simulink model "LEDLC"  (R2022b)
settings: Solver=FixedStepAuto  StartTime=0.0  StopTime=10.0  FixedStep=1  RelTol=1e-3
libraries: simulink x16
settings Model: Creator=yuzehong  LastModifiedBy=yuzehong
settings OptimizationCC: DefaultParameterBehavior=Inlined  BufferReuse=off  GlobalBufferReuse=off  ExpressionFolding=off  EnableMemcpy=off  PassReuseOutputArgsAs=Individual arguments  NoFixptDivByZeroProtection=on  EfficientFloat2IntCast=on  OptimizeDataStoreBuffers=off  BusAssignmentInplaceUpdate=off  OptimizationLevel=level0  EfficientTunableParamExpr=on
settings DebuggingCC: ParameterTunabilityLossMsg=error  UnconnectedInputMsg=warning  UnconnectedOutputMsg=warning  UnconnectedLineMsg=warning
settings ModelReferenceCC: EnableRefExpFcnMdlSchedulingChecks=on
settings SFSimCC: MATLABDynamicMemAlloc=off
settings RTWCC: Description=Embedded Coder  SystemTargetFile=ert.tlc  GenCodeOnly=on  TemplateMakefile=ert_default_tmf  DLArmComputeVersion=19.05
settings CodeAppCC: GenerateComments=off  IgnoreCustomStorageClasses=off  OperatorAnnotations=on  SimulinkDataObjDesc=on  SFDataObjDesc=on  SimulinkBlockComments=off
settings ERTTargetCC: TargetLangStandard=C99 (ISO)  GenerateSampleERTMain=on  CodeInterfacePackaging=Reusable function  InlinedParameterPlacement=NonHierarchical  ERTCustomFileTemplate=example_file_process.tlc
settings ConfigComp: DVMaxProcessTime=3600  DVTestSuiteOptimization=Auto  DVDetectOutOfBounds=on  DVSaveHarnessModel=on  DVModelReferenceHarness=on

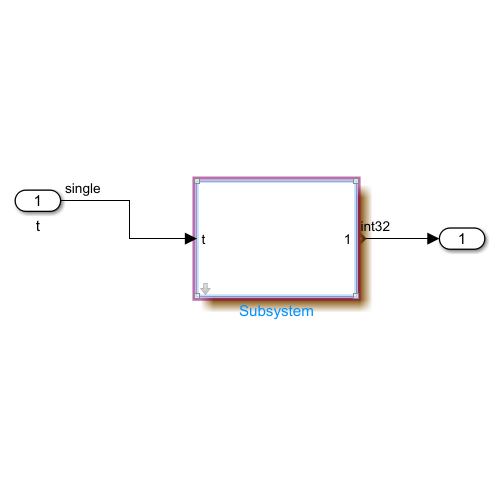
[thumbnail: Simulink's stored preview of the top-level diagram]
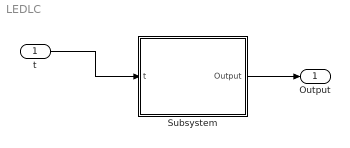
== system LEDLC ==
  t : Inport
  Subsystem : Subsystem  mask{length=64, id=3142}
      mask DialogControl ParameterGroupVar Prompt: 参数
  Output : Outport
  wires:
  t/1 -> Subsystem/1(t)
  Subsystem/1(Output) -> Output/1

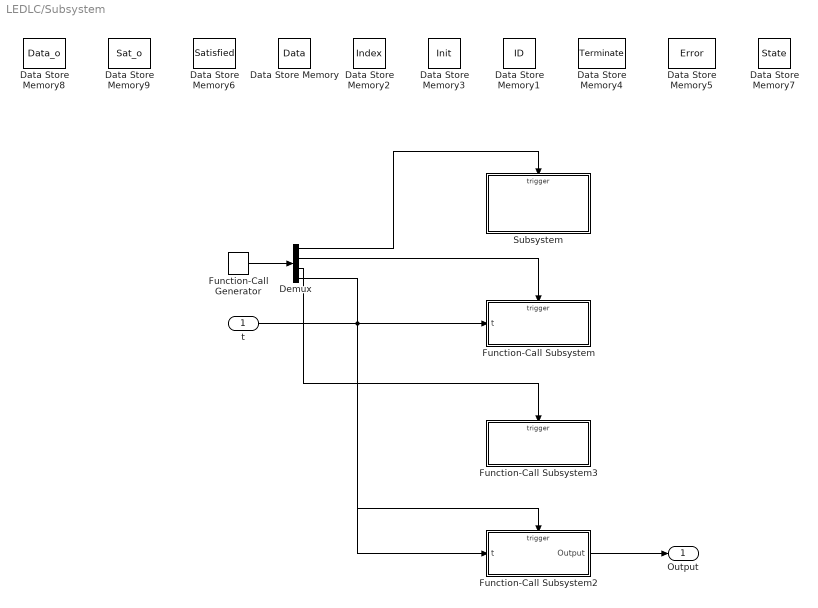
== system LEDLC/Subsystem ==
  t : Inport
  Data Store Memory : DataStoreMemory  DataStoreName=Data  WriteAfterWriteMsg=warning  ShowAdditionalParam=off  OutDataTypeStr=single  Dimensions=length
  Data Store Memory1 : DataStoreMemory  DataStoreName=ID  WriteAfterWriteMsg=warning  ShowAdditionalParam=off  OutDataTypeStr=int32
  Data Store Memory2 : DataStoreMemory  DataStoreName=Index  WriteAfterWriteMsg=warning  ShowAdditionalParam=off  OutDataTypeStr=int32
  Data Store Memory3 : DataStoreMemory  DataStoreName=Init  WriteAfterWriteMsg=warning  ShowAdditionalParam=off  OutDataTypeStr=int32
  Data Store Memory4 : DataStoreMemory  DataStoreName=Terminate  WriteAfterWriteMsg=warning  ShowAdditionalParam=off  OutDataTypeStr=int32
  Data Store Memory5 : DataStoreMemory  DataStoreName=Error  WriteAfterWriteMsg=warning  ShowAdditionalParam=off  OutDataTypeStr=int32
  Data Store Memory6 : DataStoreMemory  DataStoreName=Satisfied  WriteAfterWriteMsg=warning  ShowAdditionalParam=off  OutDataTypeStr=int32  Dimensions=length
  Data Store Memory7 : DataStoreMemory  DataStoreName=State  WriteAfterWriteMsg=warning  ShowAdditionalParam=off
  Data Store Memory8 : DataStoreMemory  DataStoreName=Data_o  WriteAfterWriteMsg=warning  ShowAdditionalParam=off  OutDataTypeStr=single  Dimensions=length
  Data Store Memory9 : DataStoreMemory  DataStoreName=Sat_o  WriteAfterWriteMsg=warning  ShowAdditionalParam=off  OutDataTypeStr=int32  Dimensions=length
  Demux : Demux
  Function-Call Generator : simulink/Ports & Subsystems/Function-Call Generator  sample_time=-1  numberOfIterations=1  DisallowWideOutput=off
  Function-Call Subsystem : Subsystem  TreatAsAtomicUnit=on
  Function-Call Subsystem2 : Subsystem  TreatAsAtomicUnit=on
  Function-Call Subsystem3 : Subsystem  TreatAsAtomicUnit=on
  Subsystem : Subsystem
  Output : Outport
  wires:
  Function-Call Generator/1 -> Demux/1
  Demux/1 -> Subsystem/Trigger
  t/1 -> Function-Call Subsystem/1(t), Function-Call Subsystem2/1(t)
  Demux/3 -> Function-Call Subsystem3/Trigger
  Function-Call Subsystem2/1(Output) -> Output/1
  Demux/4 -> Function-Call Subsystem2/Trigger
  Demux/2 -> Function-Call Subsystem/Trigger

== system LEDLC/Subsystem/Function-Call Subsystem ==
  t : Inport
  function : TriggerPort  TriggerType=function-call  VariantControl=(inherit)
  Demux : Demux  Outputs=3
  Function-Call Generator : simulink/Ports & Subsystems/Function-Call Generator  sample_time=-1  numberOfIterations=1  DisallowWideOutput=off
  Function-Call Subsystem : Subsystem  TreatAsAtomicUnit=on
  If Action Subsystem1 : Subsystem  TreatAsAtomicUnit=on
  Subsystem : Subsystem
  wires:
  Function-Call Generator/1 -> Demux/1
  Demux/3 -> If Action Subsystem1/Trigger
  Demux/1 -> Function-Call Subsystem/Trigger
  Demux/2 -> Subsystem/Trigger
  t/1 -> If Action Subsystem1/1(Inport)

== system LEDLC/Subsystem/Function-Call Subsystem2 ==
  t : Inport
  function : TriggerPort  TriggerType=function-call  VariantControl=(inherit)
  Data Store Read : DataStoreRead  DataStoreName=Terminate  IndexOptions=Index vector (dialog)  Indices=1  OutputSizes=1
  If : If  IfExpression=u1 == 0
  If Action Subsystem : Subsystem  TreatAsAtomicUnit=on
  Terminator : Terminator
  Output : Outport
  wires:
  Data Store Read/1 -> If/1
  If/1 -> Terminator/1
  If/2 -> If Action Subsystem/Action
  t/1 -> If Action Subsystem/1(t)
  If Action Subsystem/1(Output1) -> Output/1

== system LEDLC/Subsystem/Function-Call Subsystem3 ==
  function : TriggerPort  TriggerType=function-call  VariantControl=(inherit)
  Demux : Demux  Outputs=2
  Function-Call Generator : simulink/Ports & Subsystems/Function-Call Generator  sample_time=-1  numberOfIterations=1  DisallowWideOutput=off
  Function-Call Subsystem : Subsystem  TreatAsAtomicUnit=on
  Subsystem : Subsystem
  wires:
  Function-Call Generator/1 -> Demux/1
  Demux/1 -> Function-Call Subsystem/Trigger
  Demux/2 -> Subsystem/Trigger

== system LEDLC/Subsystem/Subsystem ==
  function : TriggerPort  TriggerType=function-call  VariantControl=(inherit)
  Data Store Read1 : DataStoreRead  DataStoreName=Init  IndexOptions=Index vector (dialog)  Indices=1  OutputSizes=1
  If Action Subsystem1 : Subsystem  TreatAsAtomicUnit=on
  If1 : If  IfExpression=u1 == 0
  Terminator : Terminator
  wires:
  Data Store Read1/1 -> If1/1
  If1/1 -> If Action Subsystem1/Action
  If1/2 -> Terminator/1

== system LEDLC/Subsystem/Function-Call Subsystem/Function-Call Subsystem ==
  function : TriggerPort  TriggerType=function-call  VariantControl=(inherit)
  Constant : Constant  Value=-1  OutDataTypeStr=int32
  Data Store Write : DataStoreWrite  DataStoreName=Index  IndexOptions=Index vector (dialog)  Indices=1  OutputSizes=1
  wires:
  Constant/1 -> Data Store Write/1

== system LEDLC/Subsystem/Function-Call Subsystem/If Action Subsystem1 ==
  Inport : Inport
  function : TriggerPort  TriggerType=function-call  VariantControl=(inherit)
  Data Store Read2 : DataStoreRead  DataStoreName=Index  IndexOptions=Index vector (dialog)  Indices=1  OutputSizes=1
  If : If  IfExpression=u1 ~= -1
  If Action Subsystem : Subsystem  TreatAsAtomicUnit=on
  Terminator : Terminator
  wires:
  Data Store Read2/1 -> If/1
  If/1 -> If Action Subsystem/Action
  If/2 -> Terminator/1
  Inport/1 -> If Action Subsystem/1(t)

== system LEDLC/Subsystem/Function-Call Subsystem/Subsystem ==
  function : TriggerPort  TriggerType=function-call  VariantControl=(inherit)
  For Iterator Subsystem : Subsystem  TreatAsAtomicUnit=on

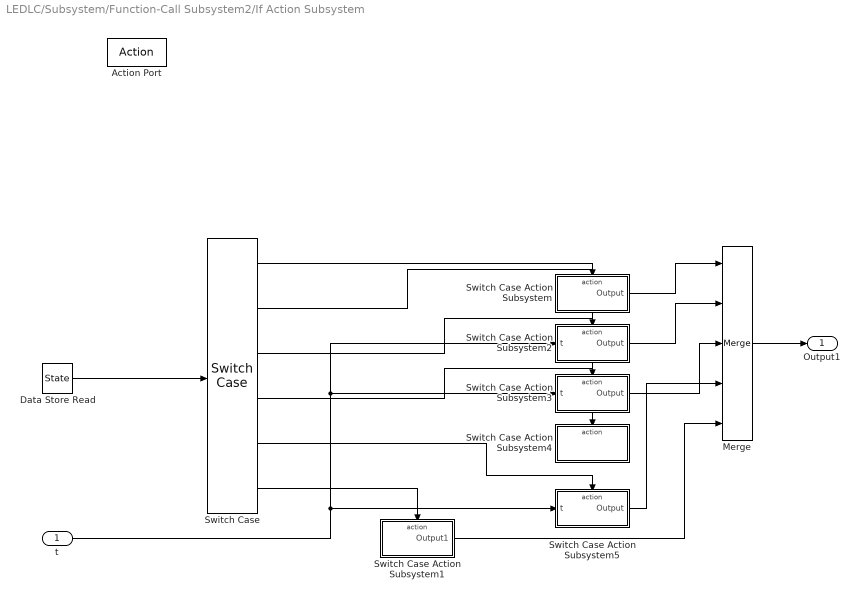
== system LEDLC/Subsystem/Function-Call Subsystem2/If Action Subsystem ==
  t : Inport
  Action Port : ActionPort  ActionPortLabel=else
  Data Store Read : DataStoreRead  DataStoreName=State  IndexOptions=Index vector (dialog)  Indices=1  OutputSizes=1
  Merge : Merge  Inputs=5
  Switch Case : SwitchCase  CaseConditions={0,1,2,3,4}
  Switch Case Action Subsystem : Subsystem  TreatAsAtomicUnit=on
  Switch Case Action Subsystem1 : Subsystem  TreatAsAtomicUnit=on
  Switch Case Action Subsystem2 : Subsystem  TreatAsAtomicUnit=on
  Switch Case Action Subsystem3 : Subsystem  TreatAsAtomicUnit=on
  Switch Case Action Subsystem4 : Subsystem  TreatAsAtomicUnit=on
  Switch Case Action Subsystem5 : Subsystem  TreatAsAtomicUnit=on
  Output1 : Outport  OutDataTypeStr=int32
  wires:
  Data Store Read/1 -> Switch Case/1
  Switch Case/1 -> Switch Case Action Subsystem/Action
  Switch Case/6 -> Switch Case Action Subsystem1/Action
  t/1 -> Switch Case Action Subsystem5/1(t), Switch Case Action Subsystem3/1(t), Switch Case Action Subsystem2/1(t)
  Switch Case/2 -> Switch Case Action Subsystem2/Action
  Switch Case Action Subsystem/1(Output) -> Merge/1
  Merge/1 -> Output1/1
  Switch Case Action Subsystem1/1(Output1) -> Merge/5
  Switch Case Action Subsystem2/1(Output) -> Merge/2
  Switch Case/3 -> Switch Case Action Subsystem3/Action
  Switch Case Action Subsystem3/1(Output) -> Merge/3
  Switch Case/4 -> Switch Case Action Subsystem4/Action
  Switch Case/5 -> Switch Case Action Subsystem5/Action
  Switch Case Action Subsystem5/1(Output) -> Merge/4

== system LEDLC/Subsystem/Function-Call Subsystem3/Function-Call Subsystem ==
  function : TriggerPort  TriggerType=function-call  VariantControl=(inherit)
  Data Store Read : DataStoreRead  DataStoreName=Terminate  IndexOptions=Index vector (dialog)  Indices=1  OutputSizes=1
  If : If
  If Action Subsystem1 : Subsystem  TreatAsAtomicUnit=on
  Terminator : Terminator
  wires:
  Data Store Read/1 -> If/1
  If/2 -> If Action Subsystem1/Action
  If/1 -> Terminator/1

== system LEDLC/Subsystem/Function-Call Subsystem3/Subsystem ==
  function : TriggerPort  TriggerType=function-call  VariantControl=(inherit)
  For Iterator Subsystem : Subsystem  TreatAsAtomicUnit=on

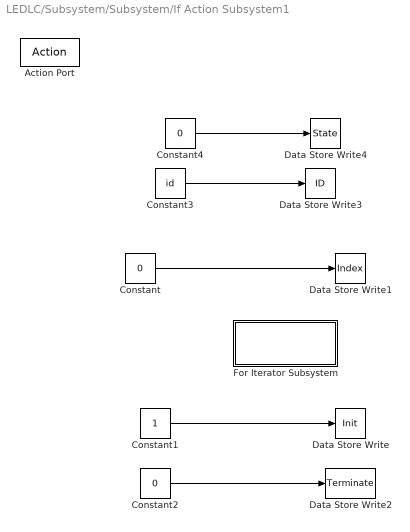
== system LEDLC/Subsystem/Subsystem/If Action Subsystem1 ==
  Action Port : ActionPort  ActionPortLabel=if(u1 == 0)
  Constant : Constant  Value=0  OutDataTypeStr=int32
  Constant1 : Constant  OutDataTypeStr=int32
  Constant2 : Constant  Value=0  OutDataTypeStr=int32
  Constant3 : Constant  Value=id  OutDataTypeStr=int32
  Constant4 : Constant  Value=0  OutDataTypeStr=int32
  Data Store Write : DataStoreWrite  DataStoreName=Init  IndexOptions=Index vector (dialog)  Indices=1  OutputSizes=1
  Data Store Write1 : DataStoreWrite  DataStoreName=Index  IndexOptions=Index vector (dialog)  Indices=1  OutputSizes=1
  Data Store Write2 : DataStoreWrite  DataStoreName=Terminate  IndexOptions=Index vector (dialog)  Indices=1  OutputSizes=1
  Data Store Write3 : DataStoreWrite  DataStoreName=ID  IndexOptions=Index vector (dialog)  Indices=1  OutputSizes=1
  Data Store Write4 : DataStoreWrite  DataStoreName=State  IndexOptions=Index vector (dialog)  Indices=1  OutputSizes=1
  For Iterator Subsystem : Subsystem  TreatAsAtomicUnit=on
  wires:
  Constant/1 -> Data Store Write1/1
  Constant1/1 -> Data Store Write/1
  Constant2/1 -> Data Store Write2/1
  Constant3/1 -> Data Store Write3/1
  Constant4/1 -> Data Store Write4/1

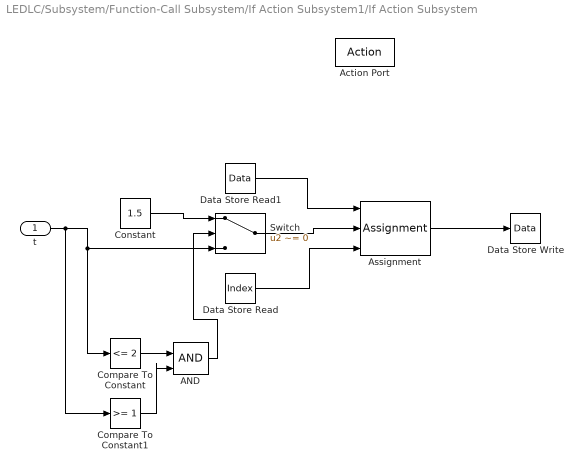
== system LEDLC/Subsystem/Function-Call Subsystem/If Action Subsystem1/If Action Subsystem ==
  t : Inport
  Action Port : ActionPort  ActionPortLabel=if(u1 ~= -1)
  AND : Logic  IconShape=distinctive  AllPortsSameDT=off  OutDataTypeStr=boolean
  Assignment : Assignment  IndexMode=Zero-based  DiagnosticForDimensions=Warning  IndexOptions=Index vector (port)  Indices=1  OutputSizes=1
  Compare To Constant : simulink/Logic and Bit Operations/Compare To Constant  relop=<=  const=2  OutDataTypeStr=boolean
  Compare To Constant1 : simulink/Logic and Bit Operations/Compare To Constant  relop=>=  const=1  OutDataTypeStr=boolean
  Constant : Constant  Value=1.5  OutDataTypeStr=single
  Data Store Read : DataStoreRead  DataStoreName=Index  IndexOptions=Index vector (dialog)  Indices=1  OutputSizes=1
  Data Store Read1 : DataStoreRead  DataStoreName=Data  IndexOptions=Index vector (dialog)  Indices=1  OutputSizes=1
  Data Store Write : DataStoreWrite  DataStoreName=Data  IndexOptions=Index vector (dialog)  Indices=1  OutputSizes=1
  Switch : Switch  Criteria=u2 ~= 0  SaturateOnIntegerOverflow=off  InputSameDT=off
  wires:
  Data Store Read1/1 -> Assignment/1
  Assignment/1 -> Data Store Write/1
  t/1 -> Compare To Constant1/1, Switch/3, Compare To Constant/1
  Data Store Read/1 -> Assignment/3
  Compare To Constant/1 -> AND/1
  Compare To Constant1/1 -> AND/2
  AND/1 -> Switch/2
  Constant/1 -> Switch/1
  Switch/1 -> Assignment/2

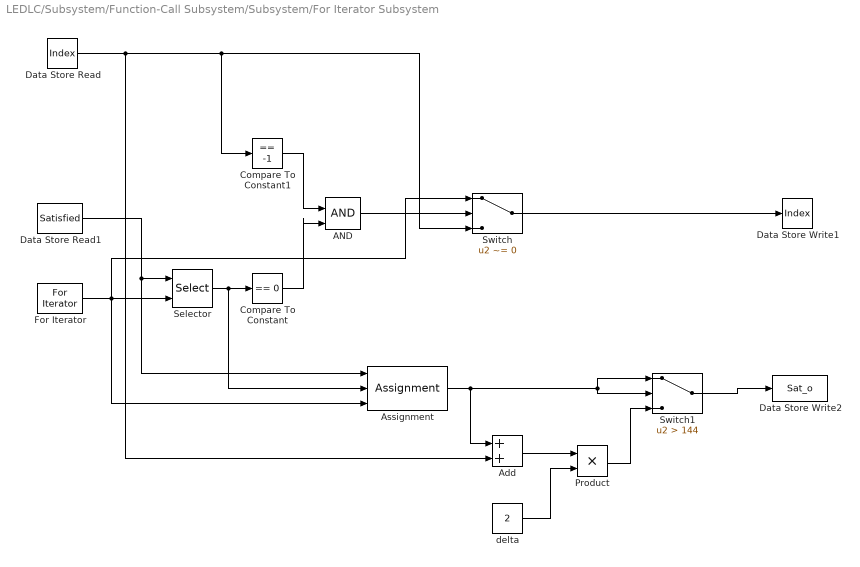
== system LEDLC/Subsystem/Function-Call Subsystem/Subsystem/For Iterator Subsystem ==
  AND : Logic  IconShape=distinctive  AllPortsSameDT=off  OutDataTypeStr=boolean
  Add : Sum  OutDataTypeStr=int32
  Assignment : Assignment  IndexMode=Zero-based  DiagnosticForDimensions=Warning  IndexOptions=Index vector (port)  Indices=1  OutputSizes=1
  Compare To Constant : simulink/Logic and Bit Operations/Compare To Constant  relop===  const=0  OutDataTypeStr=boolean
  Compare To Constant1 : simulink/Logic and Bit Operations/Compare To Constant  relop===  const=-1  OutDataTypeStr=boolean
  Data Store Read : DataStoreRead  DataStoreName=Index  IndexOptions=Index vector (dialog)  Indices=1  OutputSizes=1
  Data Store Read1 : DataStoreRead  DataStoreName=Satisfied  IndexOptions=Index vector (dialog)  Indices=1  OutputSizes=1
  Data Store Write1 : DataStoreWrite  DataStoreName=Index  IndexOptions=Index vector (dialog)  Indices=1  OutputSizes=1
  Data Store Write2 : DataStoreWrite  DataStoreName=Sat_o  IndexOptions=Index vector (dialog)  Indices=1  OutputSizes=1
  For Iterator : ForIterator  IterationLimit=length  IndexMode=Zero-based
  Product : Product  OutDataTypeStr=int32
  Selector : Selector  IndexMode=Zero-based  InputPortWidth=length  IndexOptions=Index vector (port)  Indices=[1 3]  OutputSizes=1
  Switch : Switch  Criteria=u2 ~= 0  SaturateOnIntegerOverflow=off  InputSameDT=off
  Switch1 : Switch  Criteria=u2 > Threshold  Threshold=144  SaturateOnIntegerOverflow=off  InputSameDT=off
  delta : Constant  Value=2
  wires:
  Data Store Read/1 -> Add/2, Switch/3, Compare To Constant1/1
  Data Store Read1/1 -> Assignment/1, Selector/1
  For Iterator/1 -> Assignment/3, Switch/1, Selector/2
  Selector/1 -> Assignment/2, Compare To Constant/1
  Switch/1 -> Data Store Write1/1
  Compare To Constant1/1 -> AND/1
  Compare To Constant/1 -> AND/2
  AND/1 -> Switch/2
  Assignment/1 -> Switch1/2, Switch1/1, Add/1
  Switch1/1 -> Data Store Write2/1
  Add/1 -> Product/1
  Product/1 -> Switch1/3
  delta/1 -> Product/2

== system LEDLC/Subsystem/Function-Call Subsystem2/If Action Subsystem/Switch Case Action Subsystem ==
  Action Port : ActionPort  ActionPortLabel=case [ 0 ]:
  Constant : Constant  OutDataTypeStr=int32
  Data Store Write : DataStoreWrite  DataStoreName=State  IndexOptions=Index vector (dialog)  Indices=1  OutputSizes=1
  Output : Outport  OutDataTypeStr=int32
  wires:
  Constant/1 -> Output/1, Data Store Write/1

== system LEDLC/Subsystem/Function-Call Subsystem2/If Action Subsystem/Switch Case Action Subsystem1 ==
  Action Port : ActionPort  ActionPortLabel=default:
  Constant : Constant  Value=-1  OutDataTypeStr=int32
  Output1 : Outport  OutDataTypeStr=int32
  wires:
  Constant/1 -> Output1/1

== system LEDLC/Subsystem/Function-Call Subsystem2/If Action Subsystem/Switch Case Action Subsystem2 ==
  t : Inport
  Action Port : ActionPort  ActionPortLabel=case [ 1 ]:
  If : If  IfExpression=u1 >= 2
  If Action Subsystem : Subsystem  TreatAsAtomicUnit=on
  If Action Subsystem1 : Subsystem  TreatAsAtomicUnit=on
  Merge : Merge
  Output : Outport  OutDataTypeStr=int32
  wires:
  t/1 -> If Action Subsystem/1(t), If Action Subsystem1/1(t), If/1
  Merge/1 -> Output/1
  If/2 -> If Action Subsystem1/Action
  If/1 -> If Action Subsystem/Action
  If Action Subsystem/1(Output) -> Merge/1
  If Action Subsystem1/1(Out1) -> Merge/2

== system LEDLC/Subsystem/Function-Call Subsystem2/If Action Subsystem/Switch Case Action Subsystem3 ==
  t : Inport
  Action Port : ActionPort  ActionPortLabel=case [ 2 ]:
  If : If  IfExpression=u1 > 9
  If Action Subsystem : Subsystem  TreatAsAtomicUnit=on
  If Action Subsystem1 : Subsystem  TreatAsAtomicUnit=on
  Merge : Merge
  Output : Outport  OutDataTypeStr=int32
  wires:
  t/1 -> If/1, If Action Subsystem/1(t), If Action Subsystem1/1(t)
  If/1 -> If Action Subsystem/Action
  If/2 -> If Action Subsystem1/Action
  Merge/1 -> Output/1
  If Action Subsystem/1(Output) -> Merge/1
  If Action Subsystem1/1(Out1) -> Merge/2

== system LEDLC/Subsystem/Function-Call Subsystem2/If Action Subsystem/Switch Case Action Subsystem4 ==
  Action Port : ActionPort  ActionPortLabel=case [ 3 ]:
  Constant : Constant  Value=4  OutDataTypeStr=int32
  Data Store Write : DataStoreWrite  DataStoreName=State  IndexOptions=Index vector (dialog)  Indices=1  OutputSizes=1
  wires:
  Constant/1 -> Data Store Write/1

== system LEDLC/Subsystem/Function-Call Subsystem2/If Action Subsystem/Switch Case Action Subsystem5 ==
  t : Inport
  Action Port : ActionPort  ActionPortLabel=case [ 4 ]:
  If : If  IfExpression=u1 ~= -1
  If Action Subsystem : Subsystem  TreatAsAtomicUnit=on
  Terminator : Terminator
  Output : Outport  OutDataTypeStr=int32
  wires:
  t/1 -> If Action Subsystem/1(t), If/1
  If/1 -> If Action Subsystem/Action
  If Action Subsystem/1(Output) -> Output/1
  If/2 -> Terminator/1

== system LEDLC/Subsystem/Function-Call Subsystem3/Function-Call Subsystem/If Action Subsystem1 ==
  Action Port : ActionPort  ActionPortLabel=else
  Constant : Constant  VectorParams1D=off  OutDataTypeStr=int32  SampleTime=-1
  Data Store Write : DataStoreWrite  DataStoreName=Terminate  IndexOptions=Index vector (dialog)  Indices=1  OutputSizes=1
  wires:
  Constant/1 -> Data Store Write/1

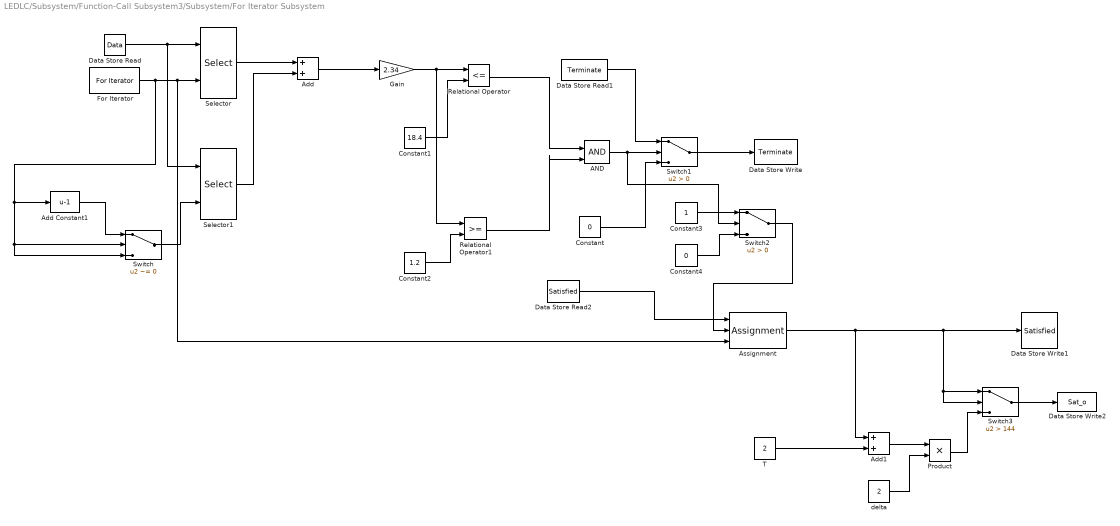
== system LEDLC/Subsystem/Function-Call Subsystem3/Subsystem/For Iterator Subsystem ==
  AND : Logic  IconShape=distinctive  AllPortsSameDT=off  OutDataTypeStr=boolean
  Add : Sum
  Add Constant1 : Bias  Bias=-1  SaturateOnIntegerOverflow=off
  Add1 : Sum  OutDataTypeStr=int32
  Assignment : Assignment  IndexMode=Zero-based  DiagnosticForDimensions=Warning  IndexOptions=Index vector (port)  Indices=1  OutputSizes=1
  Constant : Constant  Value=0  OutDataTypeStr=int32
  Constant1 : Constant  Value=18.4
  Constant2 : Constant  Value=1.2
  Constant3 : Constant  OutDataTypeStr=int32
  Constant4 : Constant  Value=0  OutDataTypeStr=int32
  Data Store Read : DataStoreRead  DataStoreName=Data  IndexOptions=Index vector (dialog)  Indices=1  OutputSizes=1
  Data Store Read1 : DataStoreRead  DataStoreName=Terminate  IndexOptions=Index vector (dialog)  Indices=1  OutputSizes=1
  Data Store Read2 : DataStoreRead  DataStoreName=Satisfied  IndexOptions=Index vector (dialog)  Indices=1  OutputSizes=1
  Data Store Write : DataStoreWrite  DataStoreName=Terminate  IndexOptions=Index vector (dialog)  Indices=1  OutputSizes=1
  Data Store Write1 : DataStoreWrite  DataStoreName=Satisfied  IndexOptions=Index vector (dialog)  Indices=1  OutputSizes=1
  Data Store Write2 : DataStoreWrite  DataStoreName=Sat_o  IndexOptions=Index vector (dialog)  Indices=1  OutputSizes=1
  For Iterator : ForIterator  IterationLimit=length  IndexMode=Zero-based
  Gain : Gain  Gain=2.34
  Product : Product  OutDataTypeStr=int32
  Relational Operator : RelationalOperator  Operator=<=  OutDataTypeStr=boolean  RndMeth=Simplest  InputSameDT=off
  Relational Operator1 : RelationalOperator  OutDataTypeStr=boolean  RndMeth=Simplest  InputSameDT=off
  Selector : Selector  IndexMode=Zero-based  InputPortWidth=length  IndexOptions=Index vector (port)  Indices=[1 3]  OutputSizes=1
  Selector1 : Selector  IndexMode=Zero-based  InputPortWidth=length  IndexOptions=Index vector (port)  Indices=[1 3]  OutputSizes=1
  Switch : Switch  Criteria=u2 ~= 0  Threshold=length-1  SaturateOnIntegerOverflow=off  InputSameDT=off
  Switch1 : Switch  Criteria=u2 > Threshold  SaturateOnIntegerOverflow=off  InputSameDT=off
  Switch2 : Switch  Criteria=u2 > Threshold  SaturateOnIntegerOverflow=off  InputSameDT=off
  Switch3 : Switch  Criteria=u2 > Threshold  Threshold=144  SaturateOnIntegerOverflow=off  InputSameDT=off
  T : Constant  Value=2
  delta : Constant  Value=2  OutDataTypeStr=int32
  wires:
  Selector/1 -> Add/1
  Add/1 -> Gain/1
  Selector1/1 -> Add/2
  Gain/1 -> Relational Operator1/1, Relational Operator/1
  Switch1/1 -> Data Store Write/1
  Constant1/1 -> Relational Operator/2
  Relational Operator/1 -> AND/1
  Data Store Read1/1 -> Switch1/1
  Constant2/1 -> Relational Operator1/2
  Relational Operator1/1 -> AND/2
  Data Store Read/1 -> Selector1/1, Selector/1
  Switch/1 -> Selector1/2
  AND/1 -> Switch2/2, Switch1/2
  Constant/1 -> Switch1/3
  Data Store Read2/1 -> Assignment/1
  Constant3/1 -> Switch2/1
  Constant4/1 -> Switch2/3
  Switch2/1 -> Assignment/2
  For Iterator/1 -> Add Constant1/1, Switch/3, Switch/2, Selector/2, Assignment/3
  Add Constant1/1 -> Switch/1
  Switch3/1 -> Data Store Write2/1
  delta/1 -> Product/2
  Product/1 -> Switch3/3
  Assignment/1 -> Add1/1, Switch3/2, Switch3/1, Data Store Write1/1
  Add1/1 -> Product/1
  T/1 -> Add1/2

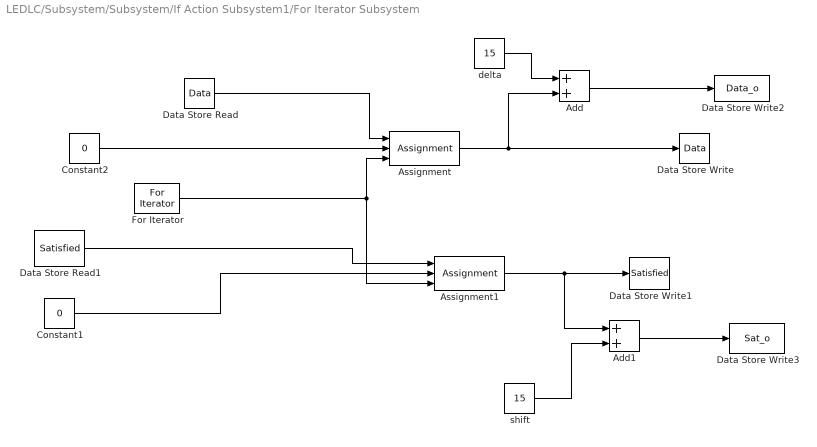
== system LEDLC/Subsystem/Subsystem/If Action Subsystem1/For Iterator Subsystem ==
  Add : Sum  OutDataTypeStr=single
  Add1 : Sum  OutDataTypeStr=int32
  Assignment : Assignment  IndexMode=Zero-based  DiagnosticForDimensions=Warning  IndexOptions=Index vector (port)  Indices=1  OutputSizes=1
  Assignment1 : Assignment  IndexMode=Zero-based  DiagnosticForDimensions=Warning  IndexOptions=Index vector (port)  Indices=1  OutputSizes=1
  Constant1 : Constant  Value=0  OutDataTypeStr=int32
  Constant2 : Constant  Value=0  OutDataTypeStr=single
  Data Store Read : DataStoreRead  DataStoreName=Data  IndexOptions=Index vector (dialog)  Indices=1  OutputSizes=1
  Data Store Read1 : DataStoreRead  DataStoreName=Satisfied  IndexOptions=Index vector (dialog)  Indices=1  OutputSizes=1
  Data Store Write : DataStoreWrite  DataStoreName=Data  IndexOptions=Index vector (dialog)  Indices=1  OutputSizes=1
  Data Store Write1 : DataStoreWrite  DataStoreName=Satisfied  IndexOptions=Index vector (dialog)  Indices=1  OutputSizes=1
  Data Store Write2 : DataStoreWrite  DataStoreName=Data_o  IndexOptions=Index vector (dialog)  Indices=1  OutputSizes=1
  Data Store Write3 : DataStoreWrite  DataStoreName=Sat_o  IndexOptions=Index vector (dialog)  Indices=1  OutputSizes=1
  For Iterator : ForIterator  IterationLimit=length  IndexMode=Zero-based
  delta : Constant  Value=15
  shift : Constant  Value=15  OutDataTypeStr=int32
  wires:
  For Iterator/1 -> Assignment1/3, Assignment/3
  Data Store Read/1 -> Assignment/1
  Assignment1/1 -> Add1/1, Data Store Write1/1
  Data Store Read1/1 -> Assignment1/1
  Constant1/1 -> Assignment1/2
  Assignment/1 -> Add/2, Data Store Write/1
  Add/1 -> Data Store Write2/1
  delta/1 -> Add/1
  Add1/1 -> Data Store Write3/1
  shift/1 -> Add1/2
  Constant2/1 -> Assignment/2

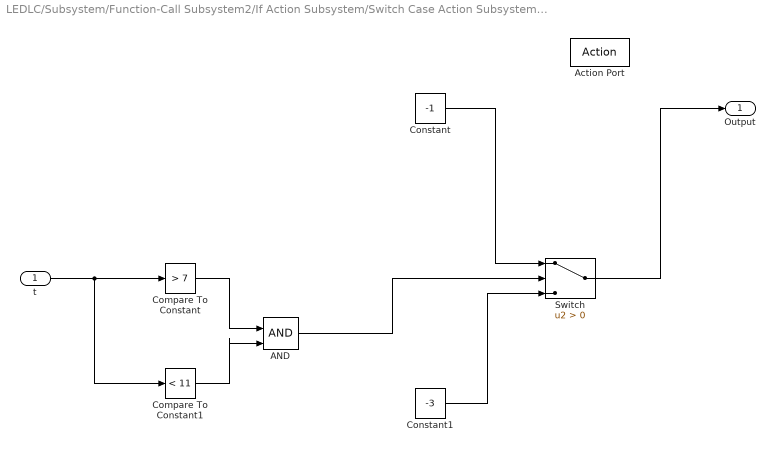
== system LEDLC/Subsystem/Function-Call Subsystem2/If Action Subsystem/Switch Case Action Subsystem2/If Action Subsystem ==
  t : Inport
  Action Port : ActionPort  ActionPortLabel=if(u1 >= 2)
  AND : Logic  IconShape=distinctive  AllPortsSameDT=off  OutDataTypeStr=boolean
  Compare To Constant : simulink/Logic and Bit Operations/Compare To Constant  relop=>  const=7  OutDataTypeStr=boolean
  Compare To Constant1 : simulink/Logic and Bit Operations/Compare To Constant  relop=<  const=11  OutDataTypeStr=boolean
  Constant : Constant  Value=-1  OutDataTypeStr=int32
  Constant1 : Constant  Value=-3  OutDataTypeStr=int32
  Switch : Switch  Criteria=u2 > Threshold  SaturateOnIntegerOverflow=off  InputSameDT=off
  Output : Outport
  wires:
  Constant/1 -> Switch/1
  t/1 -> Compare To Constant1/1, Compare To Constant/1
  Constant1/1 -> Switch/3
  Switch/1 -> Output/1
  Compare To Constant/1 -> AND/1
  Compare To Constant1/1 -> AND/2
  AND/1 -> Switch/2

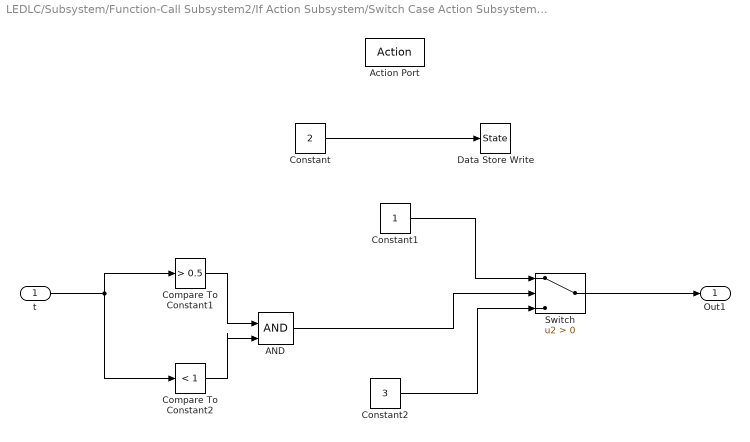
== system LEDLC/Subsystem/Function-Call Subsystem2/If Action Subsystem/Switch Case Action Subsystem2/If Action Subsystem1 ==
  t : Inport
  Action Port : ActionPort  ActionPortLabel=else
  AND : Logic  IconShape=distinctive  AllPortsSameDT=off  OutDataTypeStr=boolean
  Compare To Constant1 : simulink/Logic and Bit Operations/Compare To Constant  relop=>  const=0.5  OutDataTypeStr=boolean
  Compare To Constant2 : simulink/Logic and Bit Operations/Compare To Constant  relop=<  const=1  OutDataTypeStr=boolean
  Constant : Constant  Value=2  OutDataTypeStr=int32
  Constant1 : Constant  OutDataTypeStr=int32
  Constant2 : Constant  Value=3  OutDataTypeStr=int32
  Data Store Write : DataStoreWrite  DataStoreName=State  IndexOptions=Index vector (dialog)  Indices=1  OutputSizes=1
  Switch : Switch  Criteria=u2 > Threshold  SaturateOnIntegerOverflow=off  InputSameDT=off
  Out1 : Outport
  wires:
  Constant/1 -> Data Store Write/1
  Switch/1 -> Out1/1
  Constant1/1 -> Switch/1
  Constant2/1 -> Switch/3
  Compare To Constant2/1 -> AND/2
  Compare To Constant1/1 -> AND/1
  AND/1 -> Switch/2
  t/1 -> Compare To Constant1/1, Compare To Constant2/1

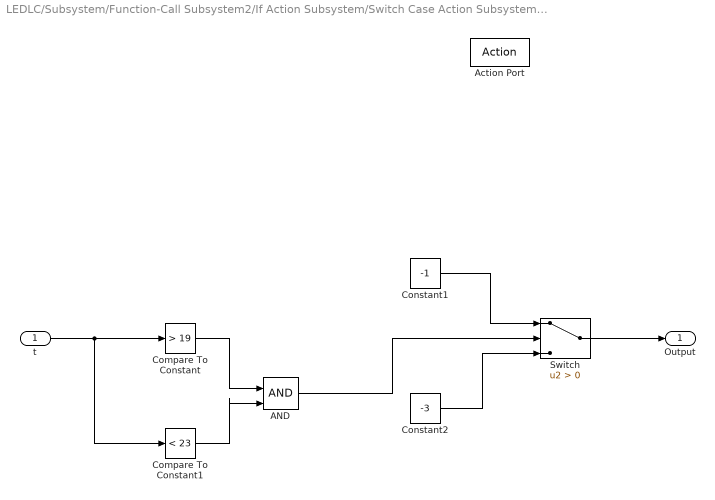
== system LEDLC/Subsystem/Function-Call Subsystem2/If Action Subsystem/Switch Case Action Subsystem3/If Action Subsystem ==
  t : Inport
  Action Port : ActionPort  ActionPortLabel=if(u1 > 9)
  AND : Logic  IconShape=distinctive  AllPortsSameDT=off  OutDataTypeStr=boolean
  Compare To Constant : simulink/Logic and Bit Operations/Compare To Constant  relop=>  const=19  OutDataTypeStr=boolean
  Compare To Constant1 : simulink/Logic and Bit Operations/Compare To Constant  relop=<  const=23  OutDataTypeStr=boolean
  Constant1 : Constant  Value=-1  OutDataTypeStr=int32
  Constant2 : Constant  Value=-3  OutDataTypeStr=int32
  Switch : Switch  Criteria=u2 > Threshold  SaturateOnIntegerOverflow=off  InputSameDT=off
  Output : Outport
  wires:
  Switch/1 -> Output/1
  Constant1/1 -> Switch/1
  Constant2/1 -> Switch/3
  Compare To Constant1/1 -> AND/2
  Compare To Constant/1 -> AND/1
  AND/1 -> Switch/2
  t/1 -> Compare To Constant1/1, Compare To Constant/1

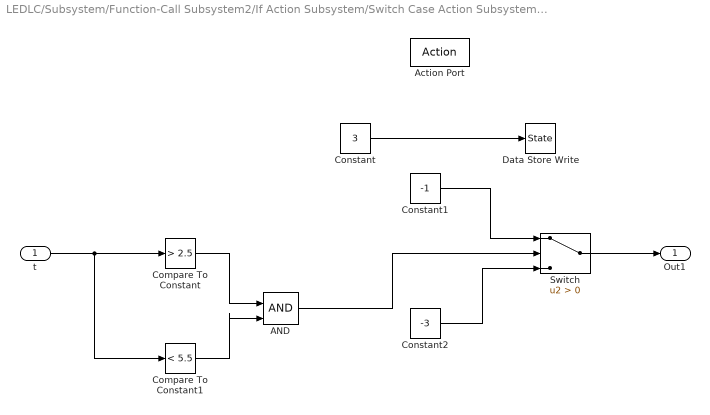
== system LEDLC/Subsystem/Function-Call Subsystem2/If Action Subsystem/Switch Case Action Subsystem3/If Action Subsystem1 ==
  t : Inport
  Action Port : ActionPort  ActionPortLabel=else
  AND : Logic  IconShape=distinctive  AllPortsSameDT=off  OutDataTypeStr=boolean
  Compare To Constant : simulink/Logic and Bit Operations/Compare To Constant  relop=>  const=2.5  OutDataTypeStr=boolean
  Compare To Constant1 : simulink/Logic and Bit Operations/Compare To Constant  relop=<  const=5.5  OutDataTypeStr=boolean
  Constant : Constant  Value=3  OutDataTypeStr=int32
  Constant1 : Constant  Value=-1  OutDataTypeStr=int32
  Constant2 : Constant  Value=-3  OutDataTypeStr=int32
  Data Store Write : DataStoreWrite  DataStoreName=State  IndexOptions=Index vector (dialog)  Indices=1  OutputSizes=1
  Switch : Switch  Criteria=u2 > Threshold  SaturateOnIntegerOverflow=off  InputSameDT=off
  Out1 : Outport
  wires:
  Constant/1 -> Data Store Write/1
  Constant2/1 -> Switch/3
  Constant1/1 -> Switch/1
  Switch/1 -> Out1/1
  Compare To Constant1/1 -> AND/2
  Compare To Constant/1 -> AND/1
  AND/1 -> Switch/2
  t/1 -> Compare To Constant1/1, Compare To Constant/1

== system LEDLC/Subsystem/Function-Call Subsystem2/If Action Subsystem/Switch Case Action Subsystem5/If Action Subsystem ==
  t : Inport
  Action Port : ActionPort  ActionPortLabel=if(u1 ~= -1)
  Compare To Constant : simulink/Logic and Bit Operations/Compare To Constant  relop=~=  const=9  OutDataTypeStr=boolean
  Constant1 : Constant  Value=-1  OutDataTypeStr=int32
  Constant2 : Constant  Value=-3  OutDataTypeStr=int32
  Switch : Switch  Criteria=u2 > Threshold  SaturateOnIntegerOverflow=off  InputSameDT=off
  Output : Outport
  wires:
  Constant2/1 -> Switch/3
  Constant1/1 -> Switch/1
  Compare To Constant/1 -> Switch/2
  Switch/1 -> Output/1
  t/1 -> Compare To Constant/1
